simulink model "main_demo_real_robot_org"  (Simulink 10.0)
settings: Solver=ode45  StartTime=0.0  StopTime=inf  RelTol=1e-3  EnableMultiTasking=on
PreLoadFcn:
  | Install_Library
StartFcn:
  | loadlibrary('ariac_vc10_i386.dll','ariac.h');
  | calllib('ariac_vc10_i386','aria_init',1,{'aria'});
  | calllib('ariac_vc10_i386','arrobot_connect');
StopFcn:
  | calllib('ariac_vc10_i386','arrobot_stop');
  | unloadlibrary ariac_vc10_i386
model workspace: external: MATLAB Code (data not in the file)
libraries: Sensors x1, Motors x1
PauseFcn:
  | calllib('ariac_vc10_i386','arrobot_stop');
ContinueFcn:
  | calllib('ariac_vc10_i386','arrobot_connect');
settings Model: Creator=Administrator  LastModifiedBy=annonymous
settings DataIOCC: LimitDataPoints=on
settings DebuggingCC: SolverPrmCheckMsg=warning  StateNameClashWarn=warning
settings GRTTargetCC: GeneratePreprocessorConditionals=Disable all  CombineOutputUpdateFcns=on  GRTInterface=off
settings ConfigComp: CovExternalEMLEnable=off

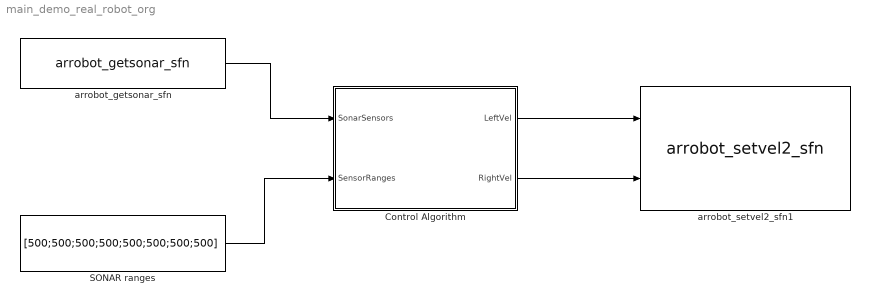
== system main_demo_real_robot_org ==
  Control Algorithm : Stateflow chart  TreatAsAtomicUnit=on  mask{v0=1}
      mask prompts: v0 "Wheel Angular Velocity"
  SONAR ranges : Constant  Value=[500;500;500;500;500;500;500;500]
  arrobot_getsonar_sfn : Sensors/arrobot_getsonar_sfn  Description=Get range readings of all front sonar on mobile robot (mm)  SFunctionSpec=void arrobot_getsonar(double y1[16])  ShowSpec=on
      settings: AttributesFormatString=Get range readings of all front sonar on mobile robot (mm)
  arrobot_setvel2_sfn1 : Motors/arrobot_setvel2_sfn  Description=Set left, right wheel velocities separately (mm/sec), overrides vel, rotvel  SFunctionSpec=void arrobot_setvel2(double u1, double u2)  ShowSpec=on
      settings: AttributesFormatString=Set left, right wheel velocities separately (mm/sec), overrides vel, rotvel
  wires:
  arrobot_getsonar_sfn/1 -> Control Algorithm/1(SonarSensors)
  Control Algorithm/1(LeftVel) -> arrobot_setvel2_sfn1/1
  Control Algorithm/2(RightVel) -> arrobot_setvel2_sfn1/2
  SONAR ranges/1 -> Control Algorithm/2(SensorRanges)

== stateflow chart Control Algorithm ==
  state Modes
    en,du:
    frontSensors = SonarSensors(4:5) < SensorRanges(4:5);
    leftMostSensors = [SonarSensors(1)] < SensorRanges(1);
    leftMiddleSensors = [SonarSensors(2:3)] < SensorRanges(2:3);
    rightMiddleSensors = [SonarSensors(6:7)] < SensorRanges(6:7);
    rightMostSensors = [SonarSensors(8) ]< SensorRanges(8);
    state ReverseABit
      en,du:
      RightVel = -v0;
      LeftVel = -v0;
    state GoStraight
      en,du:
      RightVel = v0;
      LeftVel = v0;
    state DetermineLeftRight
    state TurnRightInPlace
      du :
      RightVel = -v0;
      LeftVel = v0;
    state TurnLeftInPlace
      du :
      RightVel = v0;
      LeftVel = -v0;
    state TurnRightTight
      du :
      RightVel = v0/5;
      LeftVel = v0;
    state TurnLeftTight
      du :
      RightVel = v0;
      LeftVel = v0/5;
    state TurnRightWide
      du:
      RightVel = v0/2;
      LeftVel = v0;
    state TurnLeftWide
      du :
      RightVel = v0;
      LeftVel = v0/2;
    (default) -> ReverseABit
    ReverseABit -> GoStraight : after(3,sec)
    TurnRightWide -> GoStraight : [all(leftMostSensors<1)]
    GoStraight -> TurnRightWide [order 4] : [any(leftMostSensors>0)]
    TurnRightTight -> GoStraight : [all(leftMiddleSensors<1)]
    GoStraight -> TurnRightTight [order 2] : [any(leftMiddleSensors>0)]
    TurnRightInPlace -> GoStraight : [all(frontSensors<1)]
    GoStraight -> DetermineLeftRight [order 1] : [any(frontSensors>0)]
    TurnLeftInPlace -> GoStraight : [all(frontSensors<1)]
    TurnLeftTight -> GoStraight : [all(rightMiddleSensors<1)]
    GoStraight -> TurnLeftTight [order 3] : [any(rightMiddleSensors>0)]
    TurnLeftWide -> GoStraight : [all(rightMostSensors<1)]
    GoStraight -> TurnLeftWide [order 5] : [any(rightMostSensors>0)]
    DetermineLeftRight -> TurnRightInPlace [order 1] : [SonarSensors(4)>SonarSensors(5)]
    DetermineLeftRight -> TurnLeftInPlace [order 2] : %default
  data: LeftVel output double; RightVel output double; SonarSensors input double; frontSensors local double; SensorRanges input double; v0 parameter double; leftMostSensors local double; leftMiddleSensors local double; rightMostSensors local double; rightMiddleSensors local double
